simulink model "HighPass"  (R2022b)
settings: Solver=FixedStepDiscrete  StartTime=0.0  StopTime=10.0  RelTol=1e-3
libraries: simulink x1
settings Model: Creator=yuzehong  LastModifiedBy=yuzehong
settings OptimizationCC: DefaultParameterBehavior=Inlined  UseDivisionForNetSlopeComputation=on  GainParamInheritBuiltInType=on  UseFloatMulNetSlope=on  InlineInvariantSignals=on  PassReuseOutputArgsAs=Individual arguments  ZeroExternalMemoryAtStartup=off  ZeroInternalMemoryAtStartup=off  NoFixptDivByZeroProtection=on  EfficientFloat2IntCast=on  LifeSpan=1  OptimizeBlockOrder=speed  DifferentSizesBufferReuse=on  EfficientTunableParamExpr=on
settings DebuggingCC: ParameterTunabilityLossMsg=error
settings HardwareCC: ProdLongLongMode=on
settings SFSimCC: MATLABDynamicMemAlloc=off
settings RTWCC: Description=Embedded Coder  SystemTargetFile=ert.tlc  TemplateMakefile=ert_default_tmf
settings CodeAppCC: GenerateComments=off  IgnoreCustomStorageClasses=off  OperatorAnnotations=on  SimulinkDataObjDesc=on  SFDataObjDesc=on  CustomSymbolStrGlobalVar=rt$N$M  CustomSymbolStrType=$N$M  CustomSymbolStrFcn=$N$M$F  CustomSymbolStrMacro=$N$M  SimulinkBlockComments=off
settings ERTTargetCC: TargetLangStandard=C99 (ISO)  GenerateSampleERTMain=on  IncludeMdlTerminateFcn=off  CombineSignalStateStructs=on  SupportAbsoluteTime=off  CodeInterfacePackaging=Reusable function  SupportComplex=off  SupportNonInlinedSFcns=on  InlinedParameterPlacement=NonHierarchical  ERTCustomFileTemplate=example_file_process.tlc  ERTFilePackagingFormat=CompactWithDataFile

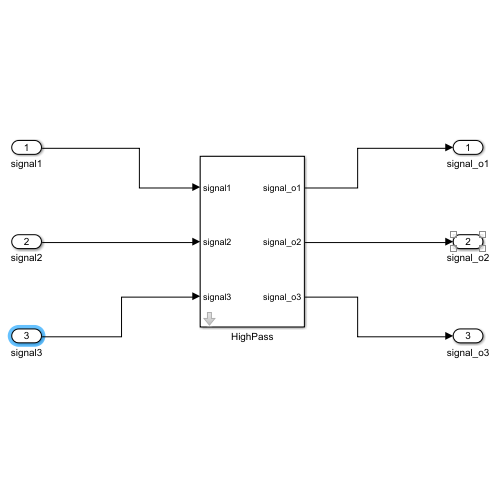
[thumbnail: Simulink's stored preview of the top-level diagram]
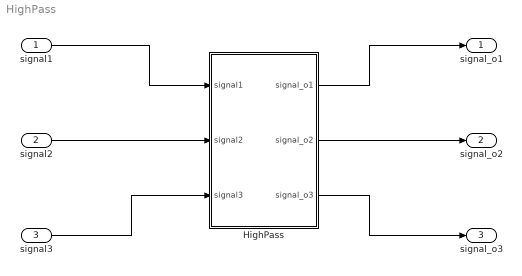
== system HighPass ==
  signal1 : Inport  PortDimensions=32
  signal2 : Inport  Port=2  PortDimensions=32
  signal3 : Inport  Port=3  PortDimensions=32
  HighPass : Subsystem  mask{length=32}
      mask DialogControl ParameterGroupVar Prompt: 参数
  signal_o1 : Outport
  signal_o2 : Outport  Port=2
  signal_o3 : Outport  Port=3
  wires:
  signal1/1 -> HighPass/1(signal1)
  signal2/1 -> HighPass/2(signal2)
  signal3/1 -> HighPass/3(signal3)
  HighPass/1(signal_o1) -> signal_o1/1
  HighPass/2(signal_o2) -> signal_o2/1
  HighPass/3(signal_o3) -> signal_o3/1

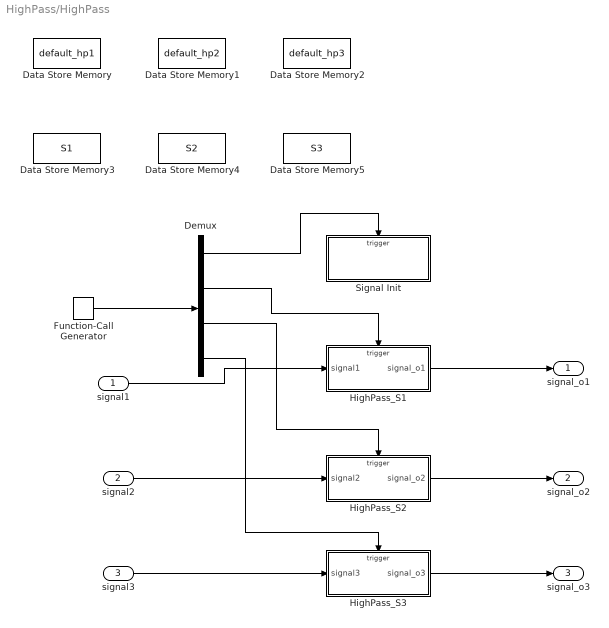
== system HighPass/HighPass ==
  signal1 : Inport  PortDimensions=length
  signal2 : Inport  Port=2  PortDimensions=length
  signal3 : Inport  Port=3  PortDimensions=length
  Data Store Memory : DataStoreMemory  DataStoreName=default_hp1  WriteAfterWriteMsg=warning  ShowAdditionalParam=off
  Data Store Memory1 : DataStoreMemory  DataStoreName=default_hp2  WriteAfterWriteMsg=warning  ShowAdditionalParam=off
  Data Store Memory2 : DataStoreMemory  DataStoreName=default_hp3  WriteAfterWriteMsg=warning  ShowAdditionalParam=off
  Data Store Memory3 : DataStoreMemory  DataStoreName=S1  WriteAfterWriteMsg=warning  ShowAdditionalParam=off  Dimensions=length
  Data Store Memory4 : DataStoreMemory  DataStoreName=S2  WriteAfterWriteMsg=warning  ShowAdditionalParam=off  Dimensions=length
  Data Store Memory5 : DataStoreMemory  DataStoreName=S3  WriteAfterWriteMsg=warning  ShowAdditionalParam=off  Dimensions=length
  Demux : Demux
  Function-Call Generator : simulink/Ports & Subsystems/Function-Call Generator  sample_time=1  numberOfIterations=1  DisallowWideOutput=off
  HighPass_S1 : Subsystem  TreatAsAtomicUnit=on
  HighPass_S2 : Subsystem  TreatAsAtomicUnit=on
  HighPass_S3 : Subsystem  TreatAsAtomicUnit=on
  Signal Init : Subsystem  TreatAsAtomicUnit=on
  signal_o1 : Outport
  signal_o2 : Outport  Port=2
  signal_o3 : Outport  Port=3
  wires:
  Function-Call Generator/1 -> Demux/1
  Demux/1 -> Signal Init/Trigger
  Demux/2 -> HighPass_S1/Trigger
  Demux/3 -> HighPass_S2/Trigger
  Demux/4 -> HighPass_S3/Trigger
  signal1/1 -> HighPass_S1/1(signal1)
  signal2/1 -> HighPass_S2/1(signal2)
  signal3/1 -> HighPass_S3/1(signal3)
  HighPass_S1/1(signal_o1) -> signal_o1/1
  HighPass_S2/1(signal_o2) -> signal_o2/1
  HighPass_S3/1(signal_o3) -> signal_o3/1

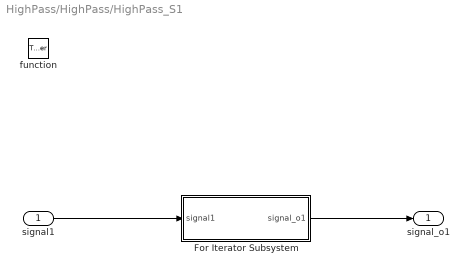
== system HighPass/HighPass/HighPass_S1 ==
  signal1 : Inport
  function : TriggerPort  TriggerType=function-call  VariantControl=(inherit)
  For Iterator Subsystem : Subsystem  TreatAsAtomicUnit=on
  signal_o1 : Outport
  wires:
  signal1/1 -> For Iterator Subsystem/1(signal1)
  For Iterator Subsystem/1(signal_o1) -> signal_o1/1

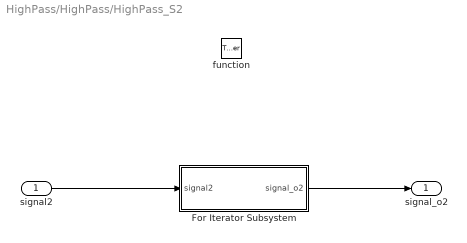
== system HighPass/HighPass/HighPass_S2 ==
  signal2 : Inport
  function : TriggerPort  TriggerType=function-call  VariantControl=(inherit)
  For Iterator Subsystem : Subsystem  TreatAsAtomicUnit=on
  signal_o2 : Outport
  wires:
  signal2/1 -> For Iterator Subsystem/1(signal2)
  For Iterator Subsystem/1(signal_o2) -> signal_o2/1

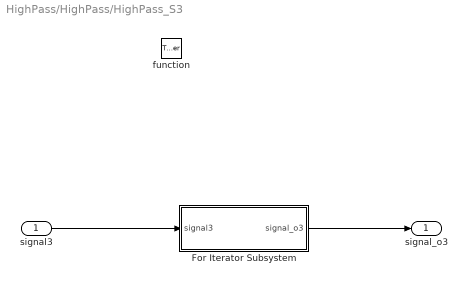
== system HighPass/HighPass/HighPass_S3 ==
  signal3 : Inport
  function : TriggerPort  TriggerType=function-call  VariantControl=(inherit)
  For Iterator Subsystem : Subsystem  TreatAsAtomicUnit=on
  signal_o3 : Outport
  wires:
  For Iterator Subsystem/1(signal_o3) -> signal_o3/1
  signal3/1 -> For Iterator Subsystem/1(signal3)

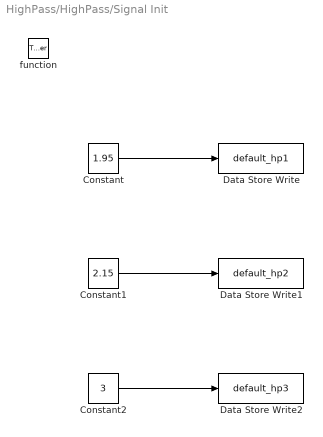
== system HighPass/HighPass/Signal Init ==
  function : TriggerPort  TriggerType=function-call  VariantControl=(inherit)
  Constant : Constant  Value=1.95  OutDataTypeStr=single
  Constant1 : Constant  Value=2.15  OutDataTypeStr=single
  Constant2 : Constant  Value=3  OutDataTypeStr=single
  Data Store Write : DataStoreWrite  DataStoreName=default_hp1  IndexOptions=Index vector (dialog)  Indices=1  OutputSizes=1
  Data Store Write1 : DataStoreWrite  DataStoreName=default_hp2  IndexOptions=Index vector (dialog)  Indices=1  OutputSizes=1
  Data Store Write2 : DataStoreWrite  DataStoreName=default_hp3  IndexOptions=Index vector (dialog)  Indices=1  OutputSizes=1
  wires:
  Constant/1 -> Data Store Write/1
  Constant1/1 -> Data Store Write1/1
  Constant2/1 -> Data Store Write2/1

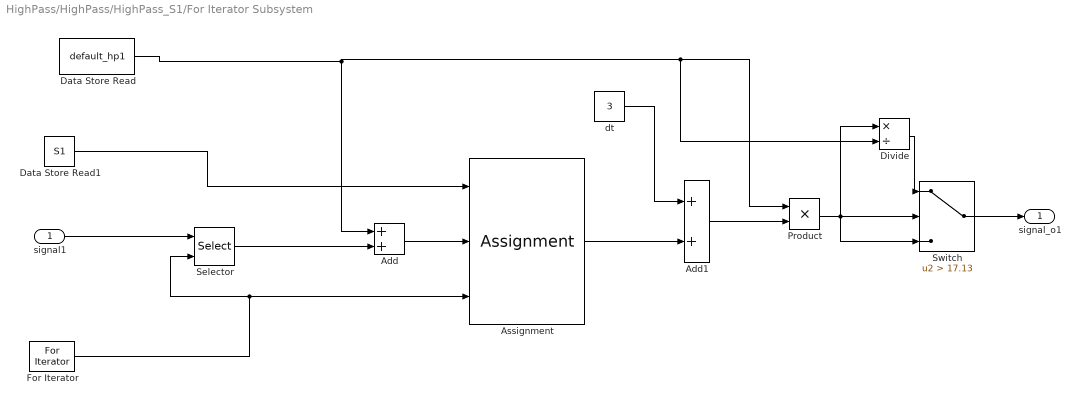
== system HighPass/HighPass/HighPass_S1/For Iterator Subsystem ==
  signal1 : Inport
  Add : Sum
  Add1 : Sum
  Assignment : Assignment  IndexMode=Zero-based  DiagnosticForDimensions=Warning  IndexOptions=Index vector (port)  Indices=1  OutputSizes=1
  Data Store Read : DataStoreRead  DataStoreName=default_hp1  IndexOptions=Index vector (dialog)  Indices=1  OutputSizes=1
  Data Store Read1 : DataStoreRead  DataStoreName=S1  IndexOptions=Index vector (dialog)  Indices=1  OutputSizes=1
  Divide : Product  Inputs=*/
  For Iterator : ForIterator  IterationLimit=length  IndexMode=Zero-based
  Product : Product
  Selector : Selector  IndexMode=Zero-based  InputPortWidth=length  IndexOptions=Index vector (port)  Indices=[1 3]  OutputSizes=1
  Switch : Switch  Criteria=u2 > Threshold  Threshold=17.13  SaturateOnIntegerOverflow=off  InputSameDT=off
  dt : Constant  Value=3
  signal_o1 : Outport
  wires:
  For Iterator/1 -> Selector/2, Assignment/3
  signal1/1 -> Selector/1
  Selector/1 -> Add/2
  Data Store Read/1 -> Add/1, Divide/2, Product/1
  Add/1 -> Assignment/2
  Assignment/1 -> Add1/2
  dt/1 -> Add1/1
  Add1/1 -> Product/2
  Product/1 -> Switch/2, Switch/3, Divide/1
  Switch/1 -> signal_o1/1
  Divide/1 -> Switch/1
  Data Store Read1/1 -> Assignment/1

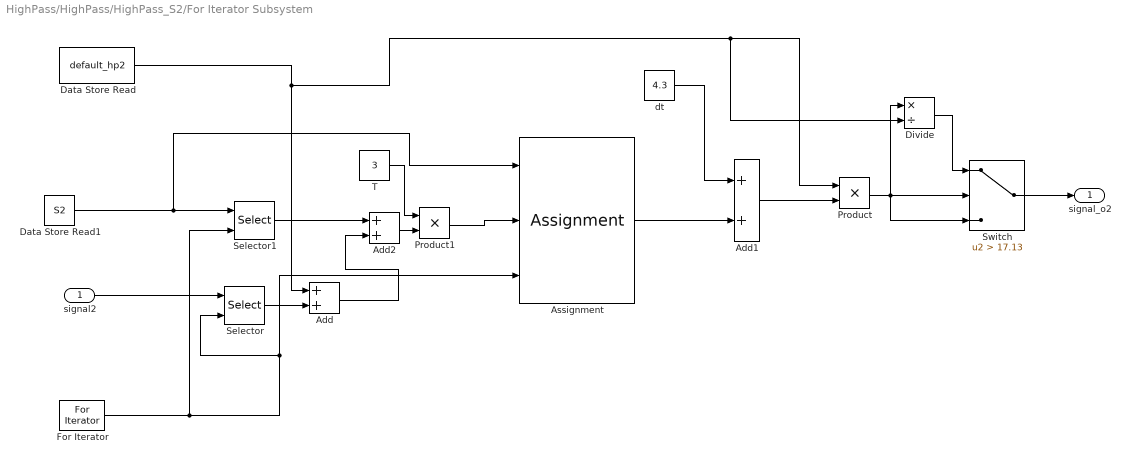
== system HighPass/HighPass/HighPass_S2/For Iterator Subsystem ==
  signal2 : Inport
  Add : Sum
  Add1 : Sum
  Add2 : Sum
  Assignment : Assignment  IndexMode=Zero-based  DiagnosticForDimensions=Warning  IndexOptions=Index vector (port)  Indices=1  OutputSizes=1
  Data Store Read : DataStoreRead  DataStoreName=default_hp2  IndexOptions=Index vector (dialog)  Indices=1  OutputSizes=1
  Data Store Read1 : DataStoreRead  DataStoreName=S2  IndexOptions=Index vector (dialog)  Indices=1  OutputSizes=1
  Divide : Product  Inputs=*/
  For Iterator : ForIterator  IterationLimit=length  IndexMode=Zero-based
  Product : Product
  Product1 : Product
  Selector : Selector  IndexMode=Zero-based  InputPortWidth=length  IndexOptions=Index vector (port)  Indices=[1 3]  OutputSizes=1
  Selector1 : Selector  IndexMode=Zero-based  InputPortWidth=length  IndexOptions=Index vector (port)  Indices=[1 3]  OutputSizes=1
  Switch : Switch  Criteria=u2 > Threshold  Threshold=17.13  SaturateOnIntegerOverflow=off  InputSameDT=off
  T : Constant  Value=3
  dt : Constant  Value=4.3
  signal_o2 : Outport
  wires:
  Assignment/1 -> Add1/2
  dt/1 -> Add1/1
  Add1/1 -> Product/2
  Product/1 -> Switch/2, Switch/3, Divide/1
  Switch/1 -> signal_o2/1
  Divide/1 -> Switch/1
  Data Store Read/1 -> Add/1, Divide/2, Product/1
  signal2/1 -> Selector/1
  For Iterator/1 -> Assignment/3, Selector/2, Selector1/2
  Add/1 -> Add2/2
  Selector1/1 -> Add2/1
  Data Store Read1/1 -> Assignment/1, Selector1/1
  Product1/1 -> Assignment/2
  Add2/1 -> Product1/2
  Selector/1 -> Add/2
  T/1 -> Product1/1

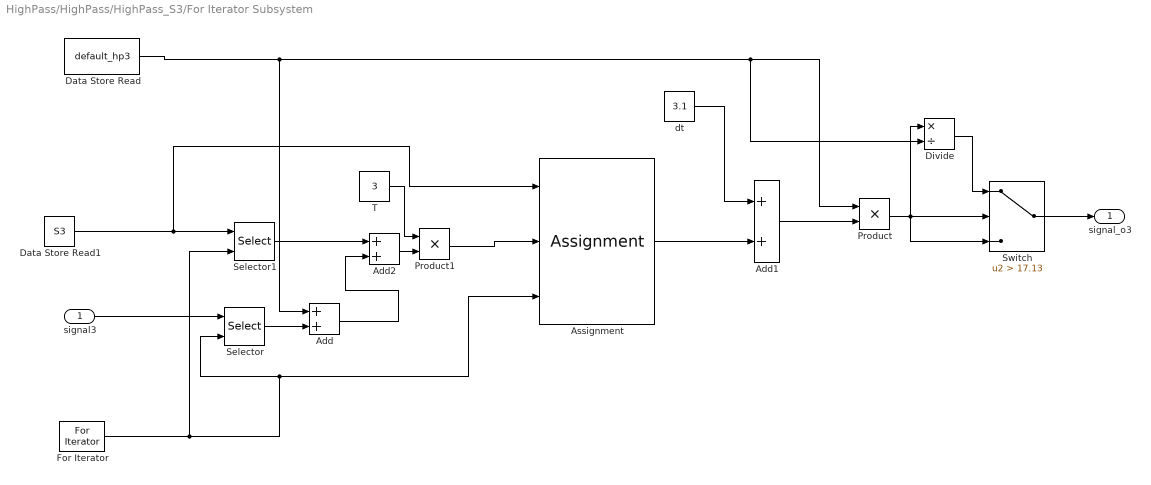
== system HighPass/HighPass/HighPass_S3/For Iterator Subsystem ==
  signal3 : Inport
  Add : Sum
  Add1 : Sum
  Add2 : Sum
  Assignment : Assignment  IndexMode=Zero-based  DiagnosticForDimensions=Warning  IndexOptions=Index vector (port)  Indices=1  OutputSizes=1
  Data Store Read : DataStoreRead  DataStoreName=default_hp3  IndexOptions=Index vector (dialog)  Indices=1  OutputSizes=1
  Data Store Read1 : DataStoreRead  DataStoreName=S3  IndexOptions=Index vector (dialog)  Indices=1  OutputSizes=1
  Divide : Product  Inputs=*/
  For Iterator : ForIterator  IterationLimit=length  IndexMode=Zero-based
  Product : Product
  Product1 : Product
  Selector : Selector  IndexMode=Zero-based  InputPortWidth=length  IndexOptions=Index vector (port)  Indices=[1 3]  OutputSizes=1
  Selector1 : Selector  IndexMode=Zero-based  InputPortWidth=length  IndexOptions=Index vector (port)  Indices=[1 3]  OutputSizes=1
  Switch : Switch  Criteria=u2 > Threshold  Threshold=17.13  SaturateOnIntegerOverflow=off  InputSameDT=off
  T : Constant  Value=3
  dt : Constant  Value=3.1
  signal_o3 : Outport
  wires:
  Assignment/1 -> Add1/2
  dt/1 -> Add1/1
  Add1/1 -> Product/2
  Product/1 -> Switch/2, Switch/3, Divide/1
  Switch/1 -> signal_o3/1
  Divide/1 -> Switch/1
  Data Store Read/1 -> Divide/2, Product/1, Add/1
  signal3/1 -> Selector/1
  For Iterator/1 -> Assignment/3, Selector/2, Selector1/2
  Add/1 -> Add2/2
  Selector1/1 -> Add2/1
  Data Store Read1/1 -> Assignment/1, Selector1/1
  Product1/1 -> Assignment/2
  Add2/1 -> Product1/2
  Selector/1 -> Add/2
  T/1 -> Product1/1
